simulink model "Relay_Test"  (R2023a)
settings: Solver=ode4  StartTime=0.0  StopTime=Tsim  FixedStep=Deltat  RelTol=1e-3
values from neighbouring files (symbols this model uses):
  Deltat = 0.05    [Test4tuner.m]
  epsilon = 0.001    [Test4tuner.m]
  Ra = 1    [Test4tuner.m]
libraries: simulink x1
settings Model: Creator=james  LastModifiedBy=james

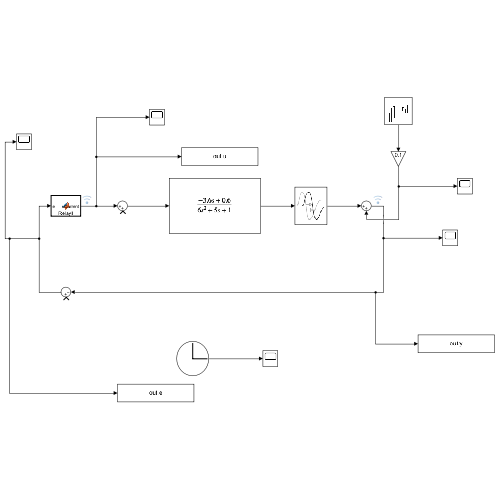
[thumbnail: Simulink's stored preview of the top-level diagram]
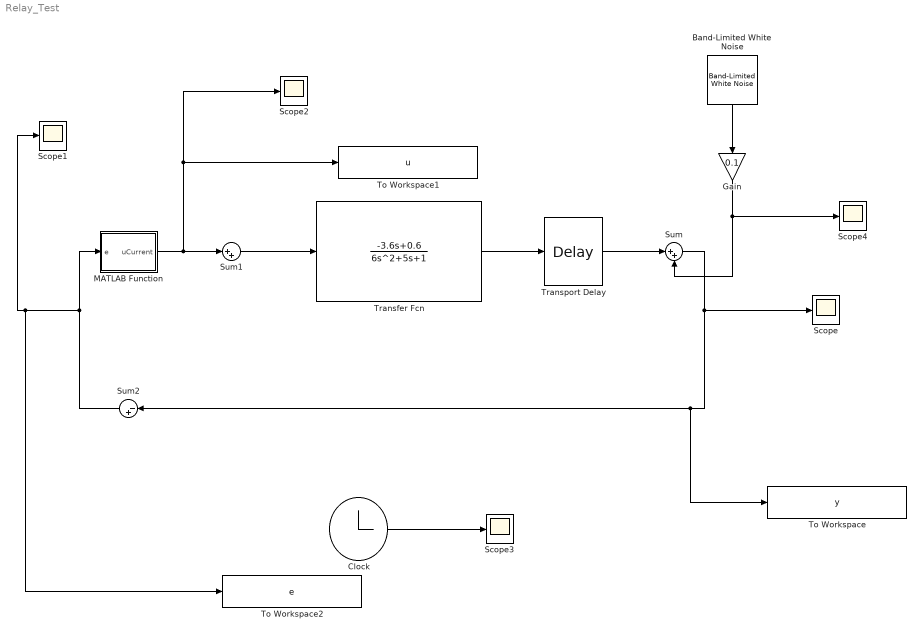
== system Relay_Test ==
  Band-Limited White Noise : simulink/Sources/Band-Limited White Noise  Cov=[1]  Ts=Deltat  seed=[23341]
  Clock : Clock
  Gain : Gain  Gain=0.1
  MATLAB Function : MATLAB Function  TreatAsAtomicUnit=on
  Scope{,1..4} (5 alike) : Scope
  Sum : Sum  Inputs=|++
  Sum1 : Sum  Inputs=|++
  Sum2 : Sum  Inputs=|-+
  To Workspace : ToWorkspace  VariableName=y  SampleTime=Deltat
  To Workspace1 : ToWorkspace  VariableName=u  SampleTime=Deltat
  To Workspace2 : ToWorkspace  VariableName=e  SampleTime=Deltat
  Transfer Fcn : TransferFcn  Numerator=[-3.6 0.6]  Denominator=[6 5 1]
  Transport Delay : TransportDelay
  wires:
  Clock/1 -> Scope3/1
  Sum/1 -> To Workspace/1, Sum2/1, Scope/1
  MATLAB Function/1(uCurrent) -> To Workspace1/1, Scope2/1, Sum1/1
  Transfer Fcn/1 -> Transport Delay/1
  Sum2/1 -> Scope1/1, To Workspace2/1, MATLAB Function/1(e)
  Sum1/1 -> Transfer Fcn/1
  Transport Delay/1 -> Sum/1
  Band-Limited White Noise/1 -> Gain/1
  Gain/1 -> Scope4/1, Sum/2

== matlab function Relay_Test/MATLAB Function ==
  settings: updateMethod=DISCRETE  sampleTime=Deltat
  data: e input; uCurrent output; epsilon parameter; Ra parameter; Deltat parameter
function uCurrent = RelayI(e,epsilon, Ra,Deltat)


persistent uPast

if isempty(uPast)

uPast = Ra;
 
end 

persistent eIPast

if isempty(eIPast)

eIPast = 0;
 
end 

eI = eIPast  + e * Deltat;

eIPast = eI;



if abs(eI) <= epsilon


    uCurrent = uPast;

else
    
    uCurrent = sign(eI) *  Ra;
    uPast = uCurrent   ;
end
